simulink library "ilcUpdate_cl"  (R2022a)
settings: Solver=VariableStepAuto  StartTime=0.0  StopTime=10.0  RelTol=1e-3
undefined symbols (not defined in the file or in its folder): ctrl
libraries: ilcUpdateLaw_cl x1, rlsGradientEst_cl x1
settings Model: Creator=mcobb  LastModifiedBy=lhill8
settings SolverCC: AlgebraicLoopSolver=TrustRegion
settings DebuggingCC: UnconnectedInputMsg=warning  UnconnectedOutputMsg=warning  UnconnectedLineMsg=warning  SFMachineParentedDataDiag=warning  ArithmeticOperatorsInVariantConditions=warning
settings SFSimCC: CustomCodeUndefinedFunction=UseInterfaceOnly

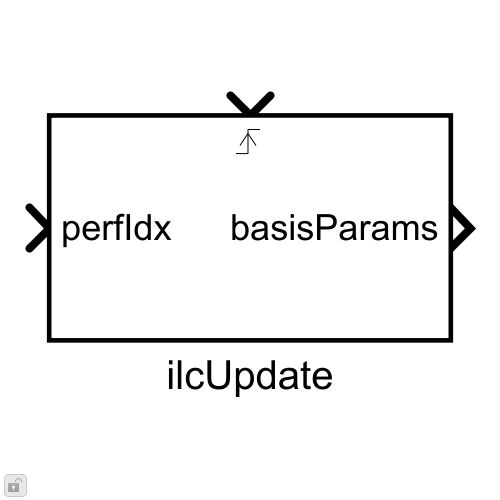
[thumbnail: Simulink's stored preview of the top-level diagram]
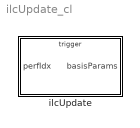
== system ilcUpdate_cl ==
  ilcUpdate : Subsystem  mask{initBasisParams=ctrl.initBasisParams.Value, lrn=ctrl.learningGain.Value, AdaptationParameter=ctrl.forgettingFactor.Value, trstRgn=0, amp=0, enableVec=0}
      mask prompts: initBasisParams "Init Basis Params"; lrn "Gradient Based Learning Gain"; AdaptationParameter "Controllib:blocks:recursiveEstimationMaskAdaptationParameterFF"; trstRgn "Trust Region Dimensions"; amp "White Noise Amplitude"; enableVec "Enable Vector"
      mask TypeOptions lrn: ilcUpdateLaw/lrn
      mask TypeOptions AdaptationParameter: rlsGradientEst/AdaptationParameter
      mask DialogControl AdaptationParameter Prompt: Forgetting Factor:

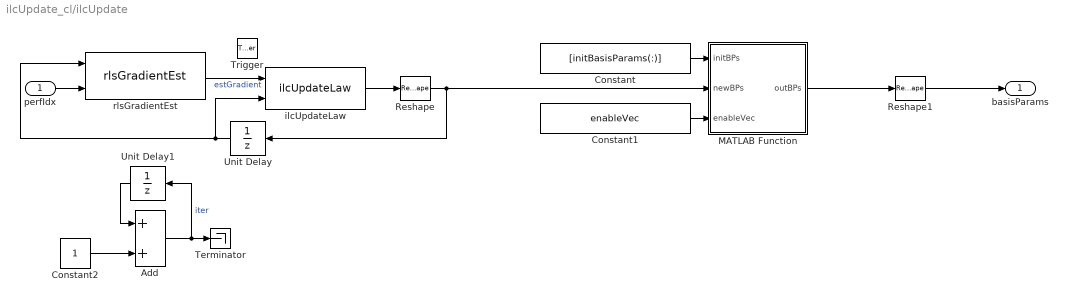
== system ilcUpdate_cl/ilcUpdate ==
  perfIdx : Inport  PortDimensions=1
  Trigger : TriggerPort  VariantControl=Variant  PortDimensions=1
  Add : Sum
  Constant : Constant  Value=[initBasisParams(:)]
  Constant1 : Constant  Value=enableVec
  Constant2 : Constant
  MATLAB Function : MATLAB Function  TreatAsAtomicUnit=on
  Reshape : Reshape
  Reshape1 : Reshape  OutputDimensionality=Column vector (2-D)
  Terminator : Terminator
  Unit Delay : UnitDelay  InitialCondition=[initBasisParams(logical(enableVec))]  SampleTime=-1  HasFrameUpgradeWarning=on
  Unit Delay1 : UnitDelay  SampleTime=-1  HasFrameUpgradeWarning=on
  ilcUpdateLaw : ilcUpdateLaw_cl/ilcUpdateLaw  lrn=lrn  trstRgn=trstRgn(logical(enableVec))  amp=amp(logical(enableVec))
  rlsGradientEst : rlsGradientEst_cl/rlsGradientEst  AdaptationParameter=AdaptationParameter  Ts=1  numParams=numel([initBasisParams(logical(enableVec))])
  basisParams : Outport  PortDimensions=[5 1]  InitialOutput=initBasisParams  VectorParamsAs1DForOutWhenUnconnected=off
  wires:
  rlsGradientEst/1 -> ilcUpdateLaw/1  "estGradient"
  perfIdx/1 -> rlsGradientEst/2
  ilcUpdateLaw/1 -> Reshape/1
  Unit Delay/1 -> rlsGradientEst/1, ilcUpdateLaw/2
  Reshape/1 -> MATLAB Function/2(newBPs), Unit Delay/1
  MATLAB Function/1(outBPs) -> Reshape1/1
  Constant/1 -> MATLAB Function/1(initBPs)
  Constant1/1 -> MATLAB Function/3(enableVec)
  Reshape1/1 -> basisParams/1
  Add/1 -> Unit Delay1/1, Terminator/1  "iter"
  Unit Delay1/1 -> Add/1
  Constant2/1 -> Add/2

== matlab function ilcUpdate_cl/ilcUpdate/MATLAB Function ==
  data: initBPs input; outBPs output; newBPs input; enableVec input
function outBPs = fcn(initBPs,newBPs,enableVec)

outBPs = initBPs;

if newBPs(1) <= newBPs(2)*2
    newBPs(2) = newBPs(1)/2-1
end
outBPs(logical(enableVec)) = newBPs;
